simulink model "smd"  (R2020b)
settings: Solver=VariableStepAuto  StartTime=0.0  StopTime=10.0  RelTol=1e-3
settings Model: Creator=divyaprakash  LastModifiedBy=divyaprakash
settings SolverCC: AlgebraicLoopSolver=LineSearch

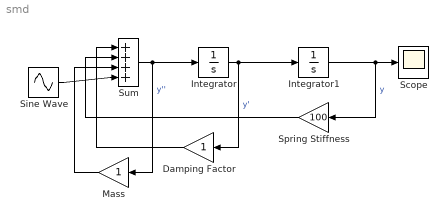
== system smd ==
  Damping Factor : Gain
  Integrator : Integrator
  Integrator1 : Integrator  InitialCondition=1
  Mass : Gain
  Scope : Scope
  Sine Wave : Sin  Amplitude=0.2  SampleTime=0
  Spring Stiffness : Gain  Gain=100
  Sum : Sum  Inputs=|++++
  wires:
  Integrator/1 -> Damping Factor/1, Integrator1/1  "y'"
  Integrator1/1 -> Spring Stiffness/1, Scope/1  "y"
  Sum/1 -> Mass/1, Integrator/1  "y''"
  Spring Stiffness/1 -> Sum/2
  Damping Factor/1 -> Sum/1
  Mass/1 -> Sum/3
  Sine Wave/1 -> Sum/4
